simulink model "pid_ai_buck_dual_loop_demo"  (R2024b)
settings: Solver=ode23t  StartTime=0.0  StopTime=0.3  MaxStep=1e-4  RelTol=1e-5
model workspace (MAT data in the model file):
  Buck_C = 0.00047
  Buck_Current_Limit = 8
  Buck_Duty_Max = 0.95
  Buck_Kii_Init = 8
  Buck_Kiv_Init = 8
  Buck_Kpi_Init = 0.04
  Buck_Kpv_Init = 0.08
  Buck_L = 0.00047
  Buck_Load_R1 = 6
  Buck_Load_R2 = 3
  Buck_Load_StepTime = 0.12
  Buck_RL = 0.08
  Buck_Vin_Disturbed = 20
  Buck_Vin_Nominal = 24
  Buck_Vin_StepTime = 0.08
  Buck_Vref = 12
libraries: slpidlib x2
settings Model: Creator=Simulink PID Agent Workbench  LastModifiedBy=27685

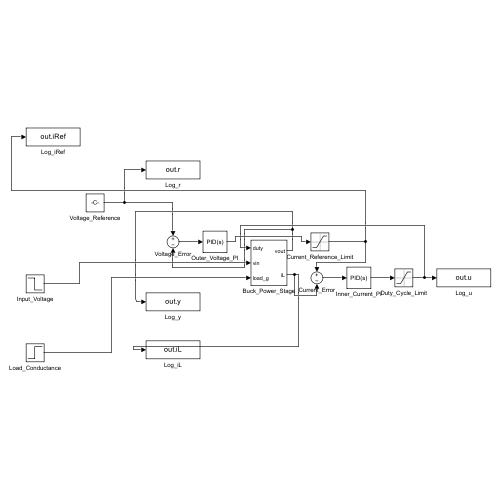
[thumbnail: Simulink's stored preview of the top-level diagram]
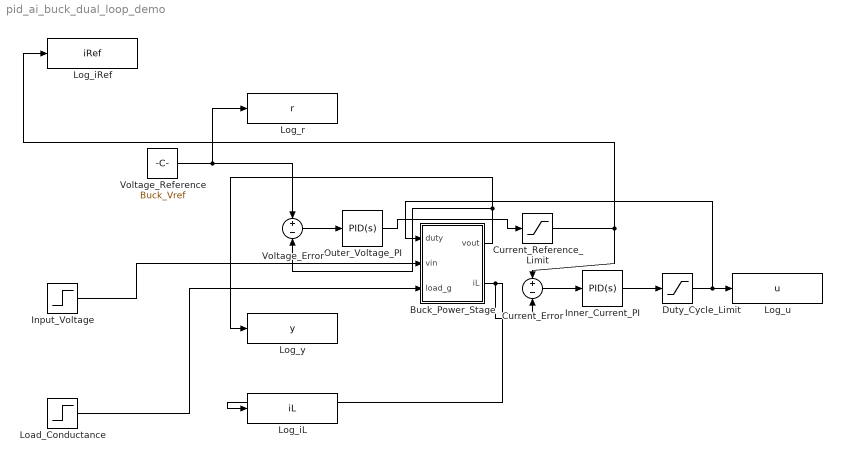
== system pid_ai_buck_dual_loop_demo ==
  Buck_Power_Stage : Subsystem
  Current_Error : Sum  Inputs=+-
  Current_Reference_Limit : Saturate  UpperLimit=Buck_Current_Limit  LowerLimit=0
  Duty_Cycle_Limit : Saturate  UpperLimit=Buck_Duty_Max  LowerLimit=0
  Inner_Current_PI : slpidlib/PID Controller  Controller=PID  Form=Parallel  TimeDomain=Continuous-time  UseExternalTs=off  SampleTime=-1  IntegratorMethod=Forward Euler  FilterMethod=Forward Euler  ControllerParametersSource=internal  P=Buck_Kpi_Init  I=Buck_Kii_Init  UseKiTs=off  D=0  UseExternalDerivativeSource=off  N=100  UseFilter=on  TunerSelectOption=Transfer Function Based (PID Tuner App)  InitialConditionSource=internal  InitialConditionForIntegrator=0  InitialConditionForFilter=0  DifferentiatorICPrevScaledInput=0  ExternalReset=none  TrackingMode=off  Kt=1  LimitOutput=off  SatLimitsSource=internal  UpperSaturationLimit=inf  LowerSaturationLimit=-inf  LinearizeAsGain=on  AntiWindupMode=none  Kb=1  LimitIntegrator=off  UpperIntegratorSaturationLimit=inf  LowerIntegratorSaturationLimit=-inf  POutMin=[]  POutMax=[]  IOutMin=[]  IOutMax=[]  DOutMin=[]  DOutMax=[]  NOutMin=[]  NOutMax=[]  SumOutMin=[]  SumOutMax=[]  SaturationOutMin=[]  SaturationOutMax=[]  PParamMin=[]  PParamMax=[]  IParamMin=[]  IParamMax=[]  DParamMin=[]  DParamMax=[]  NParamMin=[]  NParamMax=[]  KbParamMin=[]  KbParamMax=[]  KtParamMin=[]  KtParamMax=[]  KbOutMin=[]  KbOutMax=[]  KtOutMin=[]  KtOutMax=[]  IntegratorOutMin=[]  IntegratorOutMax=[]  FilterOutMin=[]  FilterOutMax=[]  SumI1OutMin=[]  SumI1OutMax=[]  SumI2OutMin=[]  SumI2OutMax=[]  SumI3OutMin=[]  SumI3OutMax=[]  SumI4OutMin=[]  SumI4OutMax=[]  SumDOutMin=[]  SumDOutMax=[]  DifferentiatorOutMin=[]  DifferentiatorOutMax=[]  FilterDiffOutCoefMin=[]  FilterDiffOutCoefMax=[]  ReciprocalOutMin=[]  ReciprocalOutMax=[]  SumDenOutMin=[]  SumDenOutMax=[]  SumNumOutMin=[]  SumNumOutMax=[]  DivideOutMin=[]  DivideOutMax=[]  UdiffTsProdOutMin=[]  UdiffTsProdOutMax=[]  NTsProdOutMin=[]  NTsProdOutMax=[]  UintegralTsProdOutMin=[]  UintegralTsProdOutMax=[]  UngainTsProdOutMin=[]  UngainTsProdOutMax=[]  ClampingZeroOutDataTypeStr=Inherit: Inherit via back propagation  ClampingZeroOutMin=[]  ClampingZeroOutMax=[]  FilterDenConstantOutDataTypeStr=Inherit: Inherit via back propagation  FilterDenConstantOutMin=[]  FilterDenConstantOutMax=[]  PCopyOutDataTypeStr=Inherit: Inherit via back propagation  PCopyOutMin=[]  PCopyOutMax=[]  NCopyOutDataTypeStr=Inherit: Inherit via back propagation  NCopyOutMin=[]  NCopyOutMax=[]  IntegratorContinuousStateAttributes=''  IntegratorStateMustResolveToSignalObject=off  IntegratorRTWStateStorageClass=Auto  FilterContinuousStateAttributes=''  FilterStateMustResolveToSignalObject=off  FilterRTWStateStorageClass=Auto  ParallelPVariant=InternalParameters  IdealPVariant=Disabled  IVariant=InternalParameters  DVariant=InternalParameters  IntegratorVariant=Continuous  SatVariant=Disabled  AWVariant=Passthrough  PCopyVariant=Disabled  TRVariant=Disabled  FdbkBlocksVariant=Forward  IdealPFdbkVariant=Disabled  SatFdbkVariant=Disabled  DerivativeFilterVariant=ContFilter  NVariant=InternalParameters  NCopyVariant=Disabled  FilterICVariant=InternalICsFilter  IntegratorICVariant=InternalICs  ExternalResetVariant=Disabled  TRSumVariant=Passthrough  SumFdbkVariant=Disabled  SumVariant=Sum_PID  TsampFilterVariant=InternalTs  TsampNgainVariant=Passthrough  TsampIntegralVariant=Disabled_SignalSpec  ExternalSaturationOutDataTypeStr=Inherit: Same as second input  DerivativeSourceVariant=ErrorSignal  PreIntVariant=InternalPreInt
  Input_Voltage : Step  Time=Buck_Vin_StepTime  Before=Buck_Vin_Nominal  After=Buck_Vin_Disturbed  SampleTime=0
  Load_Conductance : Step  Time=Buck_Load_StepTime  Before=1/Buck_Load_R1  After=1/Buck_Load_R2  SampleTime=0
  Log_iL : ToWorkspace  VariableName=iL  SaveFormat=Timeseries
  Log_iRef : ToWorkspace  VariableName=iRef  SaveFormat=Timeseries
  Log_r : ToWorkspace  VariableName=r  SaveFormat=Timeseries
  Log_u : ToWorkspace  VariableName=u  SaveFormat=Timeseries
  Log_y : ToWorkspace  VariableName=y  SaveFormat=Timeseries
  Outer_Voltage_PI : slpidlib/PID Controller  Controller=PID  Form=Parallel  TimeDomain=Continuous-time  UseExternalTs=off  SampleTime=-1  IntegratorMethod=Forward Euler  FilterMethod=Forward Euler  ControllerParametersSource=internal  P=Buck_Kpv_Init  I=Buck_Kiv_Init  UseKiTs=off  D=0  UseExternalDerivativeSource=off  N=100  UseFilter=on  TunerSelectOption=Transfer Function Based (PID Tuner App)  InitialConditionSource=internal  InitialConditionForIntegrator=0  InitialConditionForFilter=0  DifferentiatorICPrevScaledInput=0  ExternalReset=none  TrackingMode=off  Kt=1  LimitOutput=off  SatLimitsSource=internal  UpperSaturationLimit=inf  LowerSaturationLimit=-inf  LinearizeAsGain=on  AntiWindupMode=none  Kb=1  LimitIntegrator=off  UpperIntegratorSaturationLimit=inf  LowerIntegratorSaturationLimit=-inf  POutMin=[]  POutMax=[]  IOutMin=[]  IOutMax=[]  DOutMin=[]  DOutMax=[]  NOutMin=[]  NOutMax=[]  SumOutMin=[]  SumOutMax=[]  SaturationOutMin=[]  SaturationOutMax=[]  PParamMin=[]  PParamMax=[]  IParamMin=[]  IParamMax=[]  DParamMin=[]  DParamMax=[]  NParamMin=[]  NParamMax=[]  KbParamMin=[]  KbParamMax=[]  KtParamMin=[]  KtParamMax=[]  KbOutMin=[]  KbOutMax=[]  KtOutMin=[]  KtOutMax=[]  IntegratorOutMin=[]  IntegratorOutMax=[]  FilterOutMin=[]  FilterOutMax=[]  SumI1OutMin=[]  SumI1OutMax=[]  SumI2OutMin=[]  SumI2OutMax=[]  SumI3OutMin=[]  SumI3OutMax=[]  SumI4OutMin=[]  SumI4OutMax=[]  SumDOutMin=[]  SumDOutMax=[]  DifferentiatorOutMin=[]  DifferentiatorOutMax=[]  FilterDiffOutCoefMin=[]  FilterDiffOutCoefMax=[]  ReciprocalOutMin=[]  ReciprocalOutMax=[]  SumDenOutMin=[]  SumDenOutMax=[]  SumNumOutMin=[]  SumNumOutMax=[]  DivideOutMin=[]  DivideOutMax=[]  UdiffTsProdOutMin=[]  UdiffTsProdOutMax=[]  NTsProdOutMin=[]  NTsProdOutMax=[]  UintegralTsProdOutMin=[]  UintegralTsProdOutMax=[]  UngainTsProdOutMin=[]  UngainTsProdOutMax=[]  ClampingZeroOutDataTypeStr=Inherit: Inherit via back propagation  ClampingZeroOutMin=[]  ClampingZeroOutMax=[]  FilterDenConstantOutDataTypeStr=Inherit: Inherit via back propagation  FilterDenConstantOutMin=[]  FilterDenConstantOutMax=[]  PCopyOutDataTypeStr=Inherit: Inherit via back propagation  PCopyOutMin=[]  PCopyOutMax=[]  NCopyOutDataTypeStr=Inherit: Inherit via back propagation  NCopyOutMin=[]  NCopyOutMax=[]  IntegratorContinuousStateAttributes=''  IntegratorStateMustResolveToSignalObject=off  IntegratorRTWStateStorageClass=Auto  FilterContinuousStateAttributes=''  FilterStateMustResolveToSignalObject=off  FilterRTWStateStorageClass=Auto  ParallelPVariant=InternalParameters  IdealPVariant=Disabled  IVariant=InternalParameters  DVariant=InternalParameters  IntegratorVariant=Continuous  SatVariant=Disabled  AWVariant=Passthrough  PCopyVariant=Disabled  TRVariant=Disabled  FdbkBlocksVariant=Forward  IdealPFdbkVariant=Disabled  SatFdbkVariant=Disabled  DerivativeFilterVariant=ContFilter  NVariant=InternalParameters  NCopyVariant=Disabled  FilterICVariant=InternalICsFilter  IntegratorICVariant=InternalICs  ExternalResetVariant=Disabled  TRSumVariant=Passthrough  SumFdbkVariant=Disabled  SumVariant=Sum_PID  TsampFilterVariant=InternalTs  TsampNgainVariant=Passthrough  TsampIntegralVariant=Disabled_SignalSpec  ExternalSaturationOutDataTypeStr=Inherit: Same as second input  DerivativeSourceVariant=ErrorSignal  PreIntVariant=InternalPreInt
  Voltage_Error : Sum  Inputs=+-
  Voltage_Reference : Constant  Value=Buck_Vref
  wires:
  Buck_Power_Stage/2(iL) -> Current_Error/2, Log_iL/1
  Buck_Power_Stage/1(vout) -> Voltage_Error/2, Log_y/1
  Load_Conductance/1 -> Buck_Power_Stage/3(load_g)
  Input_Voltage/1 -> Buck_Power_Stage/2(vin)
  Duty_Cycle_Limit/1 -> Buck_Power_Stage/1(duty), Log_u/1
  Inner_Current_PI/1 -> Duty_Cycle_Limit/1
  Current_Error/1 -> Inner_Current_PI/1
  Current_Reference_Limit/1 -> Current_Error/1, Log_iRef/1
  Outer_Voltage_PI/1 -> Current_Reference_Limit/1
  Voltage_Error/1 -> Outer_Voltage_PI/1
  Voltage_Reference/1 -> Voltage_Error/1, Log_r/1

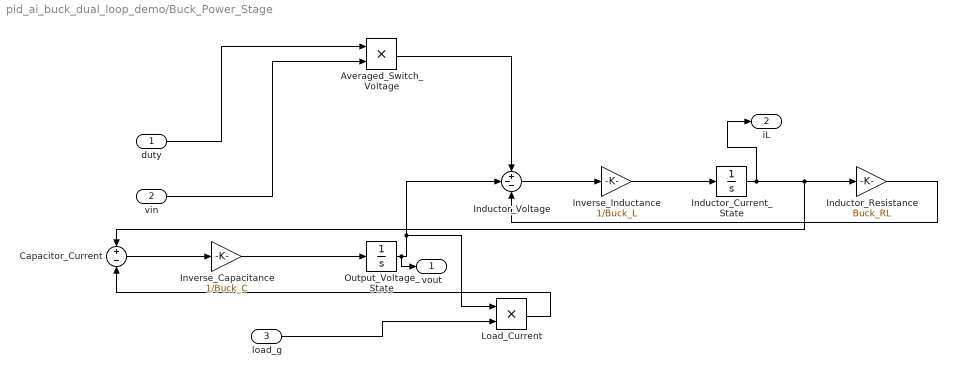
== system pid_ai_buck_dual_loop_demo/Buck_Power_Stage ==
  duty : Inport
  vin : Inport  Port=2
  load_g : Inport  Port=3
  Averaged_Switch_Voltage : Product  Inputs=**
  Capacitor_Current : Sum  Inputs=+-
  Inductor_Current_State : Integrator
  Inductor_Resistance : Gain  Gain=Buck_RL
  Inductor_Voltage : Sum  Inputs=+--
  Inverse_Capacitance : Gain  Gain=1/Buck_C
  Inverse_Inductance : Gain  Gain=1/Buck_L
  Load_Current : Product  Inputs=**
  Output_Voltage_State : Integrator
  vout : Outport
  iL : Outport  Port=2
  wires:
  Inverse_Capacitance/1 -> Output_Voltage_State/1
  Capacitor_Current/1 -> Inverse_Capacitance/1
  Load_Current/1 -> Capacitor_Current/2
  load_g/1 -> Load_Current/2
  Inverse_Inductance/1 -> Inductor_Current_State/1
  Inductor_Voltage/1 -> Inverse_Inductance/1
  Inductor_Resistance/1 -> Inductor_Voltage/3
  Inductor_Current_State/1 -> Capacitor_Current/1, Inductor_Resistance/1, iL/1
  Output_Voltage_State/1 -> Load_Current/1, Inductor_Voltage/2, vout/1
  Averaged_Switch_Voltage/1 -> Inductor_Voltage/1
  vin/1 -> Averaged_Switch_Voltage/2
  duty/1 -> Averaged_Switch_Voltage/1
